simulink model "Assem1"  (R2013a)
settings: Solver=ode45  StartTime=0.0  StopTime=50  RelTol=1e-3
undefined symbols (not defined in the file or in its folder): mass, platform, wheel
libraries: mblibv1 x14
settings Model: Creator=Raja  LastModifiedBy=Raja
settings SimMechanicsCC: VisOnUpdateDiagram=on  VisDuringSimulation=on

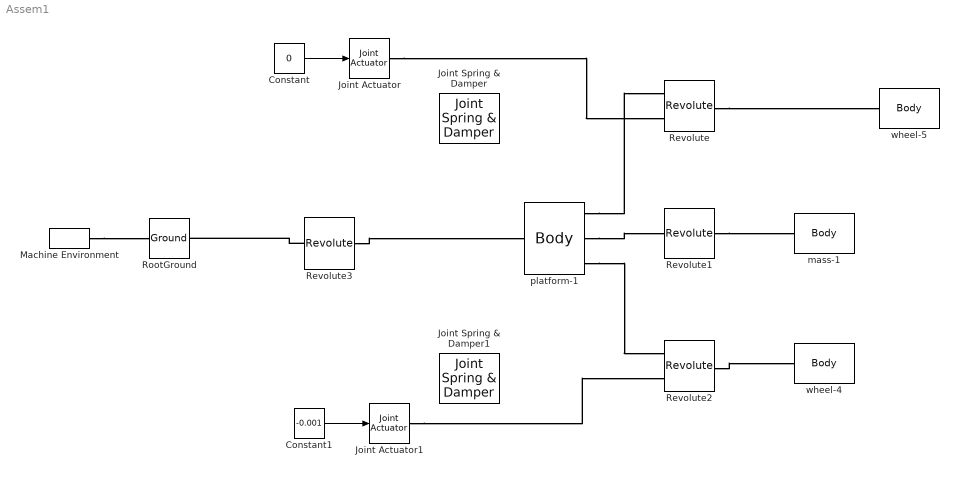
== system Assem1 ==
  Constant : Constant  Value=0
  Constant1 : Constant  Value=-0.001
  Joint Actuator : mblibv1/Sensors &  Actuators/Joint Actuator  UpdateFromCAD=off  PhysicalDomain=Mechanical  PortType=blob  ActuationStyle=Force  AngleUnits=deg  ArcVelocityUnits=deg/s  ArcAccelerationUnits=deg/s^2  CoordPositionUnits=m  VelocityUnits=m/s  AccelerationUnits=m/s^2  ForceUnits=N  TorqueUnits=N-m  ActiveIO=on  Width=1  DialogClass=MechanicalActuatorBlock  Primitive=R1  ReferenceFrame=Absolute (World)
  Joint Actuator1 : mblibv1/Sensors &  Actuators/Joint Actuator  UpdateFromCAD=off  PhysicalDomain=Mechanical  PortType=blob  ActuationStyle=Force  AngleUnits=deg  ArcVelocityUnits=deg/s  ArcAccelerationUnits=deg/s^2  CoordPositionUnits=m  VelocityUnits=m/s  AccelerationUnits=m/s^2  ForceUnits=N  TorqueUnits=N-m  ActiveIO=on  Width=1  DialogClass=MechanicalActuatorBlock  Primitive=R1  ReferenceFrame=Absolute (World)
  Joint Spring & Damper : mblibv1/Force  Elements/Joint Spring & Damper  UpdateFromCAD=off  DialogClass=JointSpringDamper  JFEParameters=P1$false$0$0$0$m$m/s$N$deg$deg/s$N*m#P2$false$0$0$0$m$m/s$N$deg$deg/s$N*m#P3$false$0$0$0$m$m/s$N$deg$deg/s$N*m#R1$true$0$0$0$m$m/s$N$deg$deg/s$N*m#R2$false$0$0$0$m$m/s$N$deg$deg/s$N*m#R3$false$0$0$0$m$m/s$N$deg$deg/s$N*m#S$false$0$0$0$m$m/s$N$deg$deg/s$N*m
  Joint Spring & Damper1 : mblibv1/Force  Elements/Joint Spring & Damper  UpdateFromCAD=off  DialogClass=JointSpringDamper  JFEParameters=P1$false$0$0$0$m$m/s$N$deg$deg/s$N*m#P2$false$0$0$0$m$m/s$N$deg$deg/s$N*m#P3$false$0$0$0$m$m/s$N$deg$deg/s$N*m#R1$true$0$0$0$m$m/s$N$deg$deg/s$N*m#R2$false$0$0$0$m$m/s$N$deg$deg/s$N*m#R3$false$0$0$0$m$m/s$N$deg$deg/s$N*m#S$false$0$0$0$m$m/s$N$deg$deg/s$N*m
  Machine Environment : mblibv1/Bodies/Machine Environment  PortType=env  PhysicalDomain=Mechanical  DialogTemplateClass=MECH.MachineEnvironment  SyncWhenCopied=off  Gravity=[0 -9.81 0]  GravityUnits=m/s^2  GravityAsSignal=off  Dimensionality=Auto-detect  AnalysisType=Forward dynamics  LinearAssemblyTolerance=1e-3  LinearAssemblyToleranceUnits=m  AngularAssemblyTolerance=1e-3  AngularAssemblyToleranceUnits=rad  ConstraintSolverType=Stabilizing  ConstraintRelTolerance=1e-4  ConstraintAbsTolerance=1e-4  UseRobustSingularityHandling=off  RedundancyAnalysisToleranceType=Automatically select tolerance  RedundancyAnalysisTolerance=1e-14  StatePerturbationType=Fixed  PerturbationSize=1e-5  VisualizeMachine=on  BodyVisualizationType=Use model default body geometries  BodyColorSelMode=Use model default  DefaultBodyColor=[1 0 0]
  Revolute : mblibv1/Joints/Revolute  LConnTagsString=__newl0|SA1  RConnTagsString=__newr0  UpdateFromCAD=on  PMImportedID=platform-1:-:wheel-5  NumSAPorts=1  CutJoint=off  MarkAsCut=off  Primitives=prismatic  PrimitiveProps=R1$World$[1,0,0]$revolute  DialogClass=JointBlock  R1Axis=[1,0,0]
  Revolute1 : mblibv1/Joints/Revolute  LConnTagsString=__newl0  RConnTagsString=__newr0  UpdateFromCAD=on  PMImportedID=mass-1:-:platform-1  NumSAPorts=0  CutJoint=off  MarkAsCut=off  Primitives=prismatic  PrimitiveProps=R1$WORLD$[0,1,0]$revolute  DialogClass=JointBlock  R1Axis=[0,1,0]
  Revolute2 : mblibv1/Joints/Revolute  LConnTagsString=__newl0|SA1  RConnTagsString=__newr0  UpdateFromCAD=on  PMImportedID=platform-1:-:wheel-4  NumSAPorts=1  CutJoint=off  MarkAsCut=off  Primitives=prismatic  PrimitiveProps=R1$World$[-1,0,0]$revolute  DialogClass=JointBlock  R1Axis=[-1,0,0]
  Revolute3 : mblibv1/Joints/Revolute  LConnTagsString=__newl0  RConnTagsString=__newr0  UpdateFromCAD=on  NumSAPorts=0  CutJoint=off  MarkAsCut=off  Primitives=prismatic  PrimitiveProps=R1$World$[1,0,0]$revolute  DialogClass=JointBlock  R1Axis=[1,0,0]
  RootGround : mblibv1/Bodies/Ground  UpdateFromCAD=on  PMImportedID=RootGround  LeftPortType=env  RightPortType=workingframe  PhysicalDomain=Mechanical  DialogClass=GroundBlock  CoordPosition=[0,0,0]  CoordPositionUnits=m  StateVectorMgrId=-1  MachineId=[0 0]  ShowEnvPort=on
  mass-1 : mblibv1/Bodies/Body  LConnTagsString=CS2  UpdateFromCAD=on  PMImportedID=mass-1  DialogClass=MechanicalBodyBlock  Mass=0.994043  MassUnits=kg  InertiaUnits=kg*m^2  Inertia=[0.000433605,0,0;0,0.000718103,0;0,0,0.000433605]  Shape=Cylinder  ShapeDims=[1 1]  ShapeUnits=m  ShapeUse=false  Density=1  DensityUnits=kg/m^3  DensityUse=false  GraphicsMode=GFXFILE  GraphicsFileName=Assem1 - mass-1.STL  BodyColorSelMode=COLORPALETTE  BodyColor=[0.647059;0.619608;0.588235]  AttachedToCS=CS1  CG=Right$CG$[0 0.515 0]$WORLD$WORLD$m$[0.837169 0 0.546944;0 -1 0;0.546944 0 -0.837169]$3x3 Transform$rad$WORLD$false$mass-1::CG(AUTOGEN)  WorkingFrames=Right$CS1$[0 0.53 0]$WORLD$WORLD$m$[0.837169 0 0.546944;0 -1 0;0.546944 0 -0.837169]$3x3 Transform$rad$WORLD$false$mass-1::CS1(AUTOGEN)#Left$CS2$[0 0.5 0]$WORLD$WORLD$m$[1 0 0;0 1 0;0 0 1]$3x3 Transform$rad$WORLD$true$mass-1:-:platform-1::mass-1(AUTOGEN)  CGPos=[0 0.515 0]  CGRot=[0.837169 0 0.546944;0 -1 0;0.546944 0 -0.837169]  CS0Pos=[]  CS0Rot=[]  CS1Pos=[0 0.53 0]  CS1Rot=[0.837169 0 0.546944;0 -1 0;0.546944 0 -0.837169]  CS2Pos=[0 0.5 0]  CS2Rot=[1 0 0;0 1 0;0 0 1]  CS3Pos=[]  CS3Rot=[]  CS4Pos=[]  CS4Rot=[]  CS5Pos=[]  CS5Rot=[]  CS6Pos=[]  CS6Rot=[]  CS7Pos=[]  CS7Rot=[]  CS8Pos=[]  CS8Rot=[]  CS9Pos=[]  CS9Rot=[]  CS10Pos=[]  CS10Rot=[]  CS11Pos=[]  CS11Rot=[]  CS12Pos=[]  CS12Rot=[]  CS13Pos=[]  CS13Rot=[]  CS14Pos=[]  CS14Rot=[]  CS15Pos=[]  CS15Rot=[]  CS16Pos=[]  CS16Rot=[]  CS17Pos=[]  CS17Rot=[]  CS18Pos=[]  CS18Rot=[]  CS19Pos=[]  CS19Rot=[]  CS20Pos=[]  CS20Rot=[]
  platform-1 : mblibv1/Bodies/Body  LConnTagsString=CS1  RConnTagsString=CS2|CS3|CS4  UpdateFromCAD=on  PMImportedID=platform-1  DialogClass=MechanicalBodyBlock  Mass=0.91444  MassUnits=kg  InertiaUnits=kg*m^2  Inertia=[0.0247914,0,0;0,0.00462358,0;0,0,0.028624]  Shape=Cylinder  ShapeDims=[1 1]  ShapeUnits=m  ShapeUse=false  Density=1  DensityUnits=kg/m^3  DensityUse=false  GraphicsMode=GFXFILE  GraphicsFileName=Assem1 - platform-1.STL  BodyColorSelMode=COLORPALETTE  BodyColor=[0.86667 0.9098 1]  AttachedToCS=CS1  CG=Right$CG$[0 0.110196 0]$WORLD$WORLD$m$[1 0 0;0 -1 0;0 0 -1]$3x3 Transform$rad$WORLD$false$platform-1::CG(AUTOGEN)  WorkingFrames=Left$CS1$[0 0 0]$WORLD$WORLD$m$[1 0 0;0 -1 0;0 0 -1]$3x3 Transform$rad$WORLD$true$platform-1::CS1(AUTOGEN)#Right$CS2$[-0.165 -0.0275 0]$WORLD$WORLD$m$[1 0 0;0 1 0;0 0 1]$3x3 Transform$rad$WORLD$true$platform-1:-:wheel-5::platform-1(AUTOGEN)#Right$CS3$[0 0.5 0]$WORLD$WORLD$m$[1 0 0;0 1 0;0 0 1]$3x3 Transform$rad$WORLD$true$mass-1:-:platform-1::platform-1(AUTOGEN)#Right$CS4$[0.165 -0.0275 0]$WORLD$WORLD$m$[1 0 0;0 1 0;0 0 1]$3x3 Transform$rad$WORLD$true$platform-1:-:wheel-4::platform-1(AUTOGEN)  CGPos=[0 0.110196 0]  CGRot=[1 0 0;0 -1 0;0 0 -1]  CS0Pos=[]  CS0Rot=[]  CS1Pos=[0 0 0]  CS1Rot=[1 0 0;0 -1 0;0 0 -1]  CS2Pos=[-0.165 -0.0275 0]  CS2Rot=[1 0 0;0 1 0;0 0 1]  CS3Pos=[0 0.5 0]  CS3Rot=[1 0 0;0 1 0;0 0 1]  CS4Pos=[0.165 -0.0275 0]  CS4Rot=[1 0 0;0 1 0;0 0 1]  CS5Pos=[]  CS5Rot=[]  CS6Pos=[]  CS6Rot=[]  CS7Pos=[]  CS7Rot=[]  CS8Pos=[]  CS8Rot=[]  CS9Pos=[]  CS9Rot=[]  CS10Pos=[]  CS10Rot=[]  CS11Pos=[]  CS11Rot=[]  CS12Pos=[]  CS12Rot=[]  CS13Pos=[]  CS13Rot=[]  CS14Pos=[]  CS14Rot=[]  CS15Pos=[]  CS15Rot=[]  CS16Pos=[]  CS16Rot=[]  CS17Pos=[]  CS17Rot=[]  CS18Pos=[]  CS18Rot=[]  CS19Pos=[]  CS19Rot=[]  CS20Pos=[]  CS20Rot=[]
  wheel-4 : mblibv1/Bodies/Body  LConnTagsString=CS2  UpdateFromCAD=on  PMImportedID=wheel-4  DialogClass=MechanicalBodyBlock  Mass=0.38285  MassUnits=kg  InertiaUnits=kg*m^2  Inertia=[0.00079034,0,0;0,0.00042234,0;0,0,0.00042234]  Shape=Cylinder  ShapeDims=[1 1]  ShapeUnits=m  ShapeUse=false  Density=1  DensityUnits=kg/m^3  DensityUse=false  GraphicsMode=GFXFILE  GraphicsFileName=Assem1 - wheel-4.STL  BodyColorSelMode=COLORPALETTE  BodyColor=[0.294118;0.294118;0.294118]  AttachedToCS=CS1  CG=Right$CG$[0.15 -0.0275 0]$WORLD$WORLD$m$[1 0 0;0 0.750115 -0.661308;0 0.661308 0.750115]$3x3 Transform$rad$WORLD$false$wheel-4::CG(AUTOGEN)  WorkingFrames=Right$CS1$[0.135 -0.0275 0]$WORLD$WORLD$m$[1 0 0;0 0.750115 -0.661308;0 0.661308 0.750115]$3x3 Transform$rad$WORLD$false$wheel-4::CS1(AUTOGEN)#Left$CS2$[0.165 -0.0275 0]$WORLD$WORLD$m$[1 0 0;0 1 0;0 0 1]$3x3 Transform$rad$WORLD$true$platform-1:-:wheel-4::wheel-4(AUTOGEN)  CGPos=[0.15 -0.0275 0]  CGRot=[1 0 0;0 0.750115 -0.661308;0 0.661308 0.750115]  CS0Pos=[]  CS0Rot=[]  CS1Pos=[0.135 -0.0275 0]  CS1Rot=[1 0 0;0 0.750115 -0.661308;0 0.661308 0.750115]  CS2Pos=[0.165 -0.0275 0]  CS2Rot=[1 0 0;0 1 0;0 0 1]  CS3Pos=[]  CS3Rot=[]  CS4Pos=[]  CS4Rot=[]  CS5Pos=[]  CS5Rot=[]  CS6Pos=[]  CS6Rot=[]  CS7Pos=[]  CS7Rot=[]  CS8Pos=[]  CS8Rot=[]  CS9Pos=[]  CS9Rot=[]  CS10Pos=[]  CS10Rot=[]  CS11Pos=[]  CS11Rot=[]  CS12Pos=[]  CS12Rot=[]  CS13Pos=[]  CS13Rot=[]  CS14Pos=[]  CS14Rot=[]  CS15Pos=[]  CS15Rot=[]  CS16Pos=[]  CS16Rot=[]  CS17Pos=[]  CS17Rot=[]  CS18Pos=[]  CS18Rot=[]  CS19Pos=[]  CS19Rot=[]  CS20Pos=[]  CS20Rot=[]
  wheel-5 : mblibv1/Bodies/Body  LConnTagsString=CS2  UpdateFromCAD=on  PMImportedID=wheel-5  DialogClass=MechanicalBodyBlock  Mass=0.38285  MassUnits=kg  InertiaUnits=kg*m^2  Inertia=[0.00079034,0,0;0,0.00042234,0;0,0,0.00042234]  Shape=Cylinder  ShapeDims=[1 1]  ShapeUnits=m  ShapeUse=false  Density=1  DensityUnits=kg/m^3  DensityUse=false  GraphicsMode=GFXFILE  GraphicsFileName=Assem1 - wheel-5.STL  BodyColorSelMode=COLORPALETTE  BodyColor=[0.294118;0.294118;0.294118]  AttachedToCS=CS1  CG=Right$CG$[-0.15 -0.0275 0]$WORLD$WORLD$m$[-1 0 0;0 0.872369 0.488847;0 0.488847 -0.872369]$3x3 Transform$rad$WORLD$false$wheel-5::CG(AUTOGEN)  WorkingFrames=Right$CS1$[-0.135 -0.0275 0]$WORLD$WORLD$m$[-1 0 0;0 0.872369 0.488847;0 0.488847 -0.872369]$3x3 Transform$rad$WORLD$false$wheel-5::CS1(AUTOGEN)#Left$CS2$[-0.165 -0.0275 0]$WORLD$WORLD$m$[1 0 0;0 1 0;0 0 1]$3x3 Transform$rad$WORLD$true$platform-1:-:wheel-5::wheel-5(AUTOGEN)  CGPos=[-0.15 -0.0275 0]  CGRot=[-1 0 0;0 0.872369 0.488847;0 0.488847 -0.872369]  CS0Pos=[]  CS0Rot=[]  CS1Pos=[-0.135 -0.0275 0]  CS1Rot=[-1 0 0;0 0.872369 0.488847;0 0.488847 -0.872369]  CS2Pos=[-0.165 -0.0275 0]  CS2Rot=[1 0 0;0 1 0;0 0 1]  CS3Pos=[]  CS3Rot=[]  CS4Pos=[]  CS4Rot=[]  CS5Pos=[]  CS5Rot=[]  CS6Pos=[]  CS6Rot=[]  CS7Pos=[]  CS7Rot=[]  CS8Pos=[]  CS8Rot=[]  CS9Pos=[]  CS9Rot=[]  CS10Pos=[]  CS10Rot=[]  CS11Pos=[]  CS11Rot=[]  CS12Pos=[]  CS12Rot=[]  CS13Pos=[]  CS13Rot=[]  CS14Pos=[]  CS14Rot=[]  CS15Pos=[]  CS15Rot=[]  CS16Pos=[]  CS16Rot=[]  CS17Pos=[]  CS17Rot=[]  CS18Pos=[]  CS18Rot=[]  CS19Pos=[]  CS19Rot=[]  CS20Pos=[]  CS20Rot=[]
  wires:
  Constant/1 -> Joint Actuator/1
  Constant1/1 -> Joint Actuator1/1
  connections:
  platform-1/RConn1 -- Revolute/LConn1
  platform-1/RConn2 -- Revolute1/LConn1
  Revolute1/RConn1 -- mass-1/LConn1
  platform-1/RConn3 -- Revolute2/LConn1
  Revolute2/RConn1 -- wheel-4/LConn1
  Machine Environment/RConn1 -- RootGround/LConn1
  Revolute3/LConn1 -- RootGround/RConn1
  Revolute3/RConn1 -- platform-1/LConn1
  Joint Actuator/RConn1 -- Revolute/LConn2
  Joint Actuator1/RConn1 -- Revolute2/LConn2
  Revolute/RConn1 -- wheel-5/LConn1
